simulink model "RCCircuit"  (R2017a)
settings: Solver=ode5  StartTime=0.0  StopTime=10  FixedStep=0.01  RelTol=1e-3  EnableMultiTasking=on
values from neighbouring files (symbols this model uses):
  C = CAP(k)    [RCCircuit_data_plot2.m]
  R = 1.8    [DesignDCMotorUsingPIDrlocusBode.m]    (also in DiscreteDesignandEquivalent.m; RCCircuit_data_plot2.m = 1; bode_mcode.m; il_zom_hae_byungsina.m)
settings Model: Creator=gyurse  LastModifiedBy=edward
settings DataIOCC: LimitDataPoints=on  SaveFormat=Array
settings OptimizationCC: LifeSpan=inf
settings DebuggingCC: UnderspecifiedInitializationDetection=Classic  MergeDetectMultiDrivingBlocksExec=none  SolverPrmCheckMsg=warning  SFUnexpectedBacktrackingDiag=warning  SFNoUnconditionalDefaultTransitionDiag=warning  SFExecutionAtInitializationDiag=none
settings HardwareCC: ProdBitPerPointer=32  ProdBitPerSizeT=32  ProdBitPerPtrDiffT=32  ProdLargestAtomicFloat=None  ProdIntDivRoundTo=Undefined  ProdEndianess=Unspecified  ProdWordSize=32  ProdHWDeviceType=32-bit Generic
settings ModelReferenceCC: PropagateSignalLabelsOutOfModel=off
settings GRTTargetCC: TargetLangStandard=C89/C90 (ANSI)  GeneratePreprocessorConditionals=Disable all
settings ConfigComp: CovMetricSettings=dw  CovHtmlReporting=on  CovSaveCumulativeToWorkspaceVar=on  CovSaveSingleToWorkspaceVar=on  CovExternalEMLEnable=off

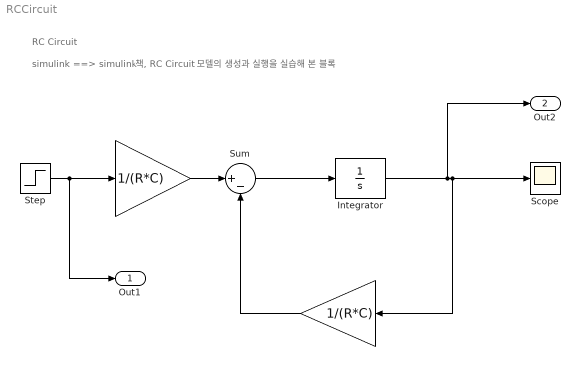
== system RCCircuit ==
  note: RC Circuit
  note: simulink ==> simulink책, RC Circuit 모델의 생성과 실행을 실습해 본 블록
  " " : Gain  Gain=1/(R*C)
  "  " : Gain  Gain=1/(R*C)
  Integrator : Integrator
  Scope : Scope
  Step : Step  Time=0  After=10  SampleTime=0
  Sum : Sum  Inputs=|+-
  Out1 : Outport
  Out2 : Outport  Port=2
  wires:
  Sum/1 -> Integrator/1
  Integrator/1 -> Out2/1, " "/1, Scope/1
  " "/1 -> Sum/2
  "  "/1 -> Sum/1
  Step/1 -> Out1/1, "  "/1
